simulink model "MMC_9lvl_matriz_tri_v12_Renner"  (R2025a)
settings: Solver=FixedStepAuto  StartTime=0.0  StopTime=5  FixedStep=0.0000005  MaxStep=1e-6  RelTol=1e-3
InitFcn:
  | C=4000e-6;
  | Larm=15e-3;
  | Rarm=0;
  | R=5;
  | L=100e-6;
  | Vcc=250;
  | Vsm=Vcc*2/4;
  | Vcap0=Vsm;
  | FR=20000;
  | TS=1/FR; %0.00005 = 50 microsec
  | Vsa=120;
  | Pref=3000;
  | Qref=0;
libraries: spsIGBTDiodeLib x48, spsVoltageMeasurementLib x34, spsSeriesRLCBranchLib x33, spsCurrentMeasurementLib x10, spsGroundLib x4, spsACVoltageSourceLib x3, SignalEditorBlockLib x2, spsDCVoltageSourceLib x2, spsPowerLib x1, sps_lib x1
(part 2 of 2)

== matlab function MMC_9lvl_matriz_tri_v12_Renner/MPC ==
  data: s1a output; s2a output; s3a output; s4a output; s5a output; s6a output; s7a output; s8a output; ioutk input; Pref input; Qref input; Ts input; R input; L input; l input; C input; Vcc input; ipn input; Vcap input; Vsm input; Vs input; s1b output; s2b output; s3b output; s4b output; s5b output; s6b output; s7b output; s8b output; s1c output; s2c output; s3c output; s4c output; s5c output; s6c output; s7c output; s8c output; ICC input; Varm input; Va output; Vb output; Vc output; Irefa output; Irefb output; Irefc output; Iza output; Izb output; Izc output
function [s1a,s2a,s3a,s4a,s5a,s6a,s7a,s8a,s1b,s2b,s3b,s4b,s5b,s6b,s7b,s8b,s1c,s2c,s3c,s4c,s5c,s6c,s7c,s8c,Va,Vb,Vc,Irefa,Irefb,Irefc,Iza,Izb,Izc]...
= MPC(ioutk,Pref, Qref,Ts,R,L,l,C,Vcc,ipn,Vcap,Vsm,Vs,ICC, Varm)

%% MATRIZ DE CHAVEAMENTOS POSSÍVEIS
    M = [0     0     0     0     0     0     0     0;
         0     0     0     0     0     0     0     1;
         0     0     0     0     0     0     1     0;
         0     0     0     0     0     0     1     1;
         0     0     0     0     0     1     0     0;
         0     0     0     0     0     1     0     1;
         0     0     0     0     0     1     1     0;
         0     0     0     0     0     1     1     1;
         0     0     0     0     1     0     0     0;
         0     0     0     0     1     0     0     1;
         0     0     0     0     1     0     1     0;
         0     0     0     0     1     0     1     1;
         0     0     0     0     1     1     0     0;
         0     0     0     0     1     1     0     1;
         0     0     0     0     1     1     1     0;
         0     0     0     0     1     1     1     1;
         0     0     0     1     0     0     0     0;
         0     0     0     1     0     0     0     1;
         0     0     0     1     0     0     1     0;
         0     0     0     1     0     0     1     1;
         0     0     0     1     0     1     0     0;
         0     0     0     1     0     1     0     1;
         0     0     0     1     0     1     1     0;
         0     0     0     1     0     1     1     1;
         0     0     0     1     1     0     0     0;
         0     0     0     1     1     0     0     1;
         0     0     0     1     1     0     1     0;
         0     0     0     1     1     0     1     1;
         0     0     0     1     1     1     0     0;
         0     0     0     1     1     1     0     1;
         0     0     0     1     1     1     1     0;
         0     0     0     1     1     1     1     1;
         0     0     1     0     0     0     0     0;
         0     0     1     0     0     0     0     1;
         0     0     1     0     0     0     1     0;
         0     0     1     0     0     0     1     1;
         0     0     1     0     0     1     0     0;
         0     0     1     0     0     1     0     1;
         0     0     1     0     0     1     1     0;
         0     0     1     0     0     1     1     1;
         0     0     1     0     1     0     0     0;
         0     0     1     0     1     0     0     1;
         0     0     1     0     1     0     1     0;
         0     0     1     0     1     0     1     1;
         0     0     1     0     1     1     0     0;
         0     0     1     0     1     1     0     1;
         0     0     1     0     1     1     1     0;
         0     0     1     0     1     1     1     1;
         0     0     1     1     0     0     0     0;
         0     0     1     1     0     0     0     1;
         0     0     1     1     0     0     1     0;
         0     0     1     1     0     0     1     1;
         0     0     1     1     0     1     0     0;
         0     0     1     1     0     1     0     1;
         0     0     1     1     0     1     1     0;
         0     0     1     1     0     1     1     1;
         0     0     1     1     1     0     0     0;
         0     0     1     1     1     0     0     1;
         0     0     1     1     1     0     1     0;
         0     0     1     1     1     0     1     1;
         0     0     1     1     1     1     0     0;
         0     0     1     1     1     1     0     1;
         0     0     1     1     1     1     1     0;
         0     0     1     1     1     1     1     1;
         0     1     0     0     0     0     0     0;
         0     1     0     0     0     0     0     1;
         0     1     0     0     0     0     1     0;
         0     1     0     0     0     0     1     1;
         0     1     0     0     0     1     0     0;
         0     1     0     0     0     1     0     1;
         0     1     0     0     0     1     1     0;
         0     1     0     0     0     1     1     1;
         0     1     0     0     1     0     0     0;
         0     1     0     0     1     0     0     1;
         0     1     0     0     1     0     1     0;
         0     1     0     0     1     0     1     1;
         0     1     0     0     1     1     0     0;
         0     1     0     0     1     1     0     1;
         0     1     0     0     1     1     1     0;
         0     1     0     0     1     1     1     1;
         0     1     0     1     0     0     0     0;
         0     1     0     1     0     0     0     1;
         0     1     0     1     0     0     1     0;
         0     1     0     1     0     0     1     1;
         0     1     0     1     0     1     0     0;
         0     1     0     1     0     1     0     1;
         0     1     0     1     0     1     1     0;
         0     1     0     1     0     1     1     1;
         0     1     0     1     1     0     0     0;
         0     1     0     1     1     0     0     1;
         0     1     0     1     1     0     1     0;
         0     1     0     1     1     0     1     1;
         0     1     0     1     1     1     0     0;
         0     1     0     1     1     1     0     1;
         0     1     0     1     1     1     1     0;
         0     1     0     1     1     1     1     1;
         0     1     1     0     0     0     0     0;
         0     1     1     0     0     0     0     1;
         0     1     1     0     0     0     1     0;
         0     1     1     0     0     0     1     1;
         0     1     1     0     0     1     0     0;
         0     1     1     0     0     1     0     1;
         0     1     1     0     0     1     1     0;
         0     1     1     0     0     1     1     1;
         0     1     1     0     1     0     0     0;
         0     1     1     0     1     0     0     1;
         0     1     1     0     1     0     1     0;
         0     1     1     0     1     0     1     1;
         0     1     1     0     1     1     0     0;
         0     1     1     0     1     1     0     1;
         0     1     1     0     1     1     1     0;
         0     1     1     0     1     1     1     1;
         0     1     1     1     0     0     0     0;
         0     1     1     1     0     0     0     1;
         0     1     1     1     0     0     1     0;
         0     1     1     1     0     0     1     1;
         0     1     1     1     0     1     0     0;
         0     1     1     1     0     1     0     1;
         0     1     1     1     0     1     1     0;
         0     1     1     1     0     1     1     1;
         0     1     1     1     1     0     0     0;
         0     1     1     1     1     0     0     1;
         0     1     1     1     1     0     1     0;
         0     1     1     1     1     0     1     1;
         0     1     1     1     1     1     0     0;
         0     1     1     1     1     1     0     1;
         0     1     1     1     1     1     1     0;
         0     1     1     1     1     1     1     1;
         1     0     0     0     0     0     0     0;
         1     0     0     0     0     0     0     1;
         1     0     0     0     0     0     1     0;
         1     0     0     0     0     0     1     1;
         1     0     0     0     0     1     0     0;
         1     0     0     0     0     1     0     1;
         1     0     0     0     0     1     1     0;
         1     0     0     0     0     1     1     1;
         1     0     0     0     1     0     0     0;
         1     0     0     0     1     0     0     1;
         1     0     0     0     1     0     1     0;
         1     0     0     0     1     0     1     1;
         1     0     0     0     1     1     0     0;
         1     0     0     0     1     1     0     1;
         1     0     0     0     1     1     1     0;
         1     0     0     0     1     1     1     1;
         1     0     0     1     0     0     0     0;
         1     0     0     1     0     0     0     1;
         1     0     0     1     0     0     1     0;
         1     0     0     1     0     0     1     1;
         1     0     0     1     0     1     0     0;
         1     0     0     1     0     1     0     1;
         1     0     0     1     0     1     1     0;
         1     0     0     1     0     1     1     1;
         1     0     0     1     1     0     0     0;
         1     0     0     1     1     0     0     1;
         1     0     0     1     1     0     1     0;
         1     0     0     1     1     0     1     1;
         1     0     0     1     1     1     0     0;
         1     0     0     1     1     1     0     1;
         1     0     0     1     1     1     1     0;
         1     0     0     1     1     1     1     1;
         1     0     1     0     0     0     0     0;
         1     0     1     0     0     0     0     1;
         1     0     1     0     0     0     1     0;
         1     0     1     0     0     0     1     1;
         1     0     1     0     0     1     0     0;
         1     0     1     0     0     1     0     1;
         1     0     1     0     0     1     1     0;
         1     0     1     0     0     1     1     1;
         1     0     1     0     1     0     0     0;
         1     0     1     0     1     0     0     1;
         1     0     1     0     1     0     1     0;
         1     0     1     0     1     0     1     1;
         1     0     1     0     1     1     0     0;
         1     0     1     0     1     1     0     1;
         1     0     1     0     1     1     1     0;
         1     0     1     0     1     1     1     1;
         1     0     1     1     0     0     0     0;
         1     0     1     1     0     0     0     1;
         1     0     1     1     0     0     1     0;
         1     0     1     1     0     0     1     1;
         1     0     1     1     0     1     0     0;
         1     0     1     1     0     1     0     1;
         1     0     1     1     0     1     1     0;
         1     0     1     1     0     1     1     1;
         1     0     1     1     1     0     0     0;
         1     0     1     1     1     0     0     1;
         1     0     1     1     1     0     1     0;
         1     0     1     1     1     0     1     1;
         1     0     1     1     1     1     0     0;
         1     0     1     1     1     1     0     1;
         1     0     1     1     1     1     1     0;
         1     0     1     1     1     1     1     1;
         1     1     0     0     0     0     0     0;
         1     1     0     0     0     0     0     1;
         1     1     0     0     0     0     1     0;
         1     1     0     0     0     0     1     1;
         1     1     0     0     0     1     0     0;
         1     1     0     0     0     1     0     1;
         1     1     0     0     0     1     1     0;
         1     1     0     0     0     1     1     1;
         1     1     0     0     1     0     0     0;
         1     1     0     0     1     0     0     1;
         1     1     0     0     1     0     1     0;
         1     1     0     0     1     0     1     1;
         1     1     0     0     1     1     0     0;
         1     1     0     0     1     1     0     1;
         1     1     0     0     1     1     1     0;
         1     1     0     0     1     1     1     1;
         1     1     0     1     0     0     0     0;
         1     1     0     1     0     0     0     1;
         1     1     0     1     0     0     1     0;
         1     1     0     1     0     0     1     1;
         1     1     0     1     0     1     0     0;
         1     1     0     1     0     1     0     1;
         1     1     0     1     0     1     1     0;
         1     1     0     1     0     1     1     1;
         1     1     0     1     1     0     0     0;
         1     1     0     1     1     0     0     1;
         1     1     0     1     1     0     1     0;
         1     1     0     1     1     0     1     1;
         1     1     0     1     1     1     0     0;
         1     1     0     1     1     1     0     1;
         1     1     0     1     1     1     1     0;
         1     1     0     1     1     1     1     1;
         1     1     1     0     0     0     0     0;
         1     1     1     0     0     0     0     1;
         1     1     1     0     0     0     1     0;
         1     1     1     0     0     0     1     1;
         1     1     1     0     0     1     0     0;
         1     1     1     0     0     1     0     1;
         1     1     1     0     0     1     1     0;
         1     1     1     0     0     1     1     1;
         1     1     1     0     1     0     0     0;
         1     1     1     0     1     0     0     1;
         1     1     1     0     1     0     1     0;
         1     1     1     0     1     0     1     1;
         1     1     1     0     1     1     0     0;
         1     1     1     0     1     1     0     1;
         1     1     1     0     1     1     1     0;
         1     1     1     0     1     1     1     1;
         1     1     1     1     0     0     0     0;
         1     1     1     1     0     0     0     1;
         1     1     1     1     0     0     1     0;
         1     1     1     1     0     0     1     1;
         1     1     1     1     0     1     0     0;
         1     1     1     1     0     1     0     1;
         1     1     1     1     0     1     1     0;
         1     1     1     1     0     1     1     1;
         1     1     1     1     1     0     0     0;
         1     1     1     1     1     0     0     1;
         1     1     1     1     1     0     1     0;
         1     1     1     1     1     0     1     1;
         1     1     1     1     1     1     0     0;
         1     1     1     1     1     1     0     1;
         1     1     1     1     1     1     1     0;
         1     1     1     1     1     1     1     1;];

%iniciando variáveis
[A,~] = size(M); %(linha,coluna)!!!!
esc=[0 0 0];
I=[0 0 0 0 0 0];
ik1=[0 0 0];
izk1=[0 0 0];
S = [0 0 0 0 0 0 0 0 0 0 0 0 0 0 0 0 0 0 0 0 0 0 0 0];
Igref = [0 0 0];
nsm=[0 0 0 0 0 0];
Vcap1 = [0 0 0 0 0 0 0 0 0 0 0 0 0 0 0 0 0 0 0 0 0 0 0 0];

kc = 1;
ki = 5;
kz = 1;

Va = (Varm(2)-Varm(1))/2; %output do bloco
Vb = (Varm(4)-Varm(3))/2;
Vc = (Varm(6)-Varm(5))/2;

Valpha = sqrt(2/3)*(Vs(1) - Vs(2)*(1/2) - Vs(3)*(1/2));
Vbeta = sqrt(2/3)*(Vs(2)*sqrt(3)*(1/2) - Vs(3)*sqrt(3)*(1/2));

Irefalpha = (Valpha*Pref + Vbeta*Qref)/(Valpha^2 + Vbeta^2);
Irefbeta = (Vbeta*Pref - Valpha*Qref)/(Valpha^2 + Vbeta^2);

Igref(1) = sqrt(2/3)*Irefalpha;
Igref(2) = sqrt(2/3)*(-Irefalpha/2 + Irefbeta*sqrt(3)/2);
Igref(3) = sqrt(2/3)*(-Irefalpha/2 - Irefbeta*sqrt(3)/2);

Irefa=Igref(1); %output do bloco
Irefb=Igref(2);
Irefc=Igref(3);

Iza = (ipn(1)+ipn(2))/2 -ICC/3;
Izb = (ipn(3)+ipn(4))/2 -ICC/3;
Izc = (ipn(5)+ipn(6))/2 -ICC/3;

%escolhendo um chaveamento com base em uma função de custo
for j  = 1:1:3
    k = (j-1)*8;
    min = inf;
    for i = 1:1:A %A é o tamanho da matriz
        Vpk1 = M(i,1)*Vcap(1+k) + M(i,2)*Vcap(2+k) + M(i,3)*Vcap(3+k) + M(i,4)*Vcap(4+k);
        Vnk1 = M(i,5)*Vcap(5+k) + M(i,6)*Vcap(6+k) + M(i,7)*Vcap(7+k) + M(i,8)*Vcap(8+k);
        
        ik1(j) = ((Vnk1-Vpk1)*(1/2) - Vs(j) + ioutk(j)*(L+l/2)/Ts)/(R+(L+l/2)/Ts);%próxima I_out_a
        izk1(j) = (ipn(1+(j-1)*2)+ipn(2+(j-1)*2))/2 -(ipn(1)+ipn(3)+ipn(5))/3 + Ts/(2*l)*(2*Vcc-Vnk1-Vpk1);%próxima I_z_a
        % izk1(j) = (ipn(1+(j-1)*2)+ipn(2+(j-1)*2))/2 -ICC/3 + Ts/(2*l)*(2*Vcc-Vnk1-Vpk1);

        Vcap1(1+k) = Vcap(1+k) + (Ts/C)*(ipn(1+(j-1)*2)*M(i,1));
        Vcap1(2+k) = Vcap(2+k) + (Ts/C)*(ipn(1+(j-1)*2)*M(i,2));
        Vcap1(3+k) = Vcap(3+k) + (Ts/C)*(ipn(1+(j-1)*2)*M(i,3));
        Vcap1(4+k) = Vcap(4+k) + (Ts/C)*(ipn(1+(j-1)*2)*M(i,4));

        Vcap1(5+k) = Vcap(5+k) + (Ts/C)*(ipn(2+(j-1)*2)*M(i,5));
        Vcap1(6+k) = Vcap(6+k) + (Ts/C)*(ipn(2+(j-1)*2)*M(i,6));
        Vcap1(7+k) = Vcap(7+k) + (Ts/C)*(ipn(2+(j-1)*2)*M(i,7));
        Vcap1(8+k) = Vcap(8+k) + (Ts/C)*(ipn(2+(j-1)*2)*M(i,8));

        g = ki*(Igref(j)-ik1(j))^4 + kz*(izk1(j))^2 + kc*(Vsm - (Vcap1(1+k)+Vcap1(2+k)+Vcap1(3+k)+Vcap1(4+k)+Vcap1(5+k)+Vcap1(6+k)+Vcap1(7+k)+Vcap1(8+k))/8)^2;
        % g = ki*(Igref(j)-ik1(j))^2 + kz*(izk1(j))^2 + kc*((Vsm - Vcap1(1+k))^2 + (Vsm - Vcap1(2+k))^2 + (Vsm - Vcap1(3+k))^2 + (Vsm - Vcap1(4+k))^2 + (Vsm - Vcap1(5+k))^2 + (Vsm - Vcap1(6+k))^2 + (Vsm - Vcap1(7+k))^2 + (Vsm - Vcap1(8+k))^2);
        % g = ki*(Igref(j)-ik1(j))^2 + kz*(izk1(j))^2 + kc*((Vsm - Vcap1(1+k))^4+ (Vsm - Vcap1(2+k))^4 + (Vsm - Vcap1(3+k))^4 + (Vsm - Vcap1(4+k))^4 + (Vsm - Vcap1(5+k))^4 + (Vsm - Vcap1(6+k))^4 + (Vsm - Vcap1(7+k))^4 + (Vsm - Vcap1(8+k))^4);
  
        if g < min
            min = g;
            esc(j) = i;
            I(j)=ik1(j);
            I(j+1)=ik1(j);
            %repetido porque eu tenho que ter essa leitura pra cada um dos
            %braços pra usar alí embaixo.
        end
    end
end

%balanceamento de capacitores

nsm(1) = M(esc(1),1) + M(esc(1),2) + M(esc(1),3) + M(esc(1),4);
nsm(2) = M(esc(1),5) + M(esc(1),6) + M(esc(1),7) + M(esc(1),8);

nsm(3) = M(esc(2),1) + M(esc(2),2) + M(esc(2),3) + M(esc(2),4);
nsm(4) = M(esc(2),5) + M(esc(2),6) + M(esc(2),7) + M(esc(2),8);

nsm(5) = M(esc(3),1) + M(esc(3),2) + M(esc(3),3) + M(esc(3),4);
nsm(6) = M(esc(3),5) + M(esc(3),6) + M(esc(3),7) + M(esc(3),8);

for j = 1:6
    k = 4 * (j - 1);
    arm_Vcap = Vcap1((1:4) + k);
    S((1:4) + k) = 0;

        if I(j) >= 0
            [~, idx] = sort(arm_Vcap, 'ascend');
        else
            [~, idx] = sort(arm_Vcap, 'descend');
        end
        selec_idx = idx(1:nsm(j));
        S(selec_idx + k) = 1;
end

S(1)=M(esc(1),1);
S(2)=M(esc(1),2);
S(3)=M(esc(1),3);
S(4)=M(esc(1),4);
S(5)=M(esc(1),5);
S(6)=M(esc(1),6);
S(7)=M(esc(1),7);
S(8)=M(esc(1),8);
S(9)=M(esc(2),1);
S(10)=M(esc(2),2);
S(11)=M(esc(2),3);
S(12)=M(esc(2),4);
S(13)=M(esc(2),5);
S(14)=M(esc(2),6);
S(15)=M(esc(2),7);
S(16)=M(esc(2),8);
S(17)=M(esc(3),1);
S(18)=M(esc(3),2);
S(19)=M(esc(3),3);
S(20)=M(esc(3),4);
S(21)=M(esc(3),5);
S(22)=M(esc(3),6);
S(23)=M(esc(3),7);
S(24)=M(esc(3),8);

% s1a=M(esc(1),1);
% s2a=M(esc(1),2);
% s3a=M(esc(1),3);
% s4a=M(esc(1),4);
% s5a=M(esc(1),5);
% s6a=M(esc(1),6);
% s7a=M(esc(1),7);
% s8a=M(esc(1),8);
% s1b=M(esc(2),1);
% s2b=M(esc(2),2);
% s3b=M(esc(2),3);
% s4b=M(esc(2),4);
% s5b=M(esc(2),5);
% s6b=M(esc(2),6);
% s7b=M(esc(2),7);
% s8b=M(esc(2),8);
% s1c=M(esc(3),1);
% s2c=M(esc(3),2);
% s3c=M(esc(3),3);
% s4c=M(esc(3),4);
% s5c=M(esc(3),5);
% s6c=M(esc(3),6);
% s7c=M(esc(3),7);
% s8c=M(esc(3),8);


s1a=S(1);
s2a=S(2);
s3a=S(3);
s4a=S(4);
s5a=S(5);
s6a=S(6);
s7a=S(7);
s8a=S(8);
s1b=S(9);
s2b=S(10);
s3b=S(11);
s4b=S(12);
s5b=S(13);
s6b=S(14);
s7b=S(15);
s8b=S(16);
s1c=S(17);
s2c=S(18);
s3c=S(19);
s4c=S(20);
s5c=S(21);
s6c=S(22);
s7c=S(23);
s8c=S(24);
